simulink model "Aufgabe2_c"  (R2020a)
settings: Solver=VariableStepAuto  StartTime=0.0  StopTime=5  RelTol=1e-9
undefined symbols (not defined in the file or in its folder): a0, b0, bf, bp, F
settings Model: Creator=seife  LastModifiedBy=seife

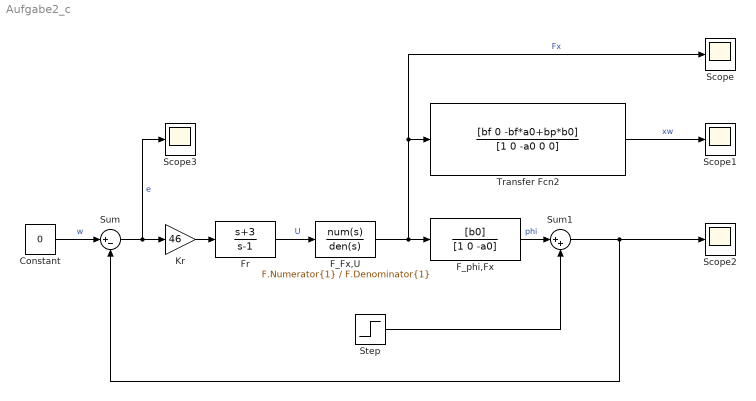
== system Aufgabe2_c ==
  Constant : Constant  Value=0
  F_Fx,U : TransferFcn  Numerator=F.Numerator{1}  Denominator=F.Denominator{1}
  F_phi,Fx : TransferFcn  Numerator=[b0]  Denominator=[1 0 -a0]
  Fr : TransferFcn  Numerator=[1 3]  Denominator=[1 -1]
  Kr : Gain  Gain=46
  Scope{,1..3} (4 alike) : Scope
  Step : Step  After=0.017  SampleTime=0
  Sum : Sum  Inputs=|+-
  Sum1 : Sum  Inputs=|++
  Transfer Fcn2 : TransferFcn  Numerator=[bf 0 -bf*a0+bp*b0]  Denominator=[1 0 -a0 0 0]
  wires:
  Transfer Fcn2/1 -> Scope1/1  "xw"
  Sum/1 -> Scope3/1, Kr/1  "e"
  Fr/1 -> F_Fx,U/1  "U"
  Constant/1 -> Sum/1  "w"
  F_phi,Fx/1 -> Sum1/1  "phi"
  Sum1/1 -> Scope2/1, Sum/2
  Kr/1 -> Fr/1
  F_Fx,U/1 -> Scope/1, Transfer Fcn2/1, F_phi,Fx/1  "Fx"
  Step/1 -> Sum1/2
